simulink model "motor_position_ctrl"  (R2020b)
settings: Solver=ode15s  StartTime=0.0  StopTime=0.2  RelTol=1e-3  AbsTol=1e-7
undefined symbols (not defined in the file): Kd, Ki, Kp, N
settings Model: DataDictionary=motor_pos_data.sldd  Creator=ADMIN  LastModifiedBy=ADMIN

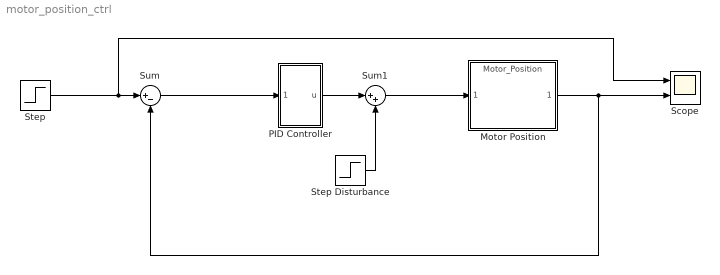
== system motor_position_ctrl ==
  "Motor Position " : ModelReference  ModelNameDialog=Motor_Position  ModelReferenceVersion=1.9
  PID Controller : Subsystem
  Scope : Scope  NumInputPorts=2
  Step : Step  Time=0  SampleTime=0
  Step Disturbance : Step  Time=0  SampleTime=0
  Sum : Sum  Inputs=|+-  SaturateOnIntegerOverflow=on
  Sum1 : Sum  Inputs=|++
  wires:
  Step/1 -> Scope/1, Sum/1
  "Motor Position "/1 -> Scope/2, Sum/2
  Sum/1 -> PID Controller/1(error)
  PID Controller/1(u) -> Sum1/1
  Sum1/1 -> "Motor Position "/1
  Step Disturbance/1 -> Sum1/2

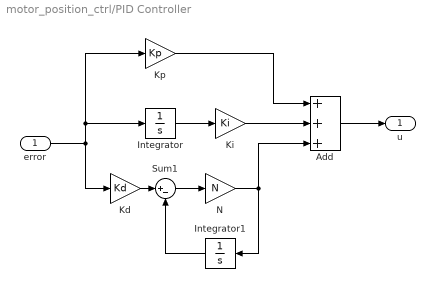
== system motor_position_ctrl/PID Controller ==
  error : Inport
  Add : Sum  Inputs=+++  SaturateOnIntegerOverflow=on
  Integrator : Integrator
  Integrator1 : Integrator
  Kd : Gain  Gain=Kd
  Ki : Gain  Gain=Ki
  Kp : Gain  Gain=Kp
  N : Gain  Gain=N
  Sum1 : Sum  Inputs=|+-
  u : Outport
  wires:
  error/1 -> Kp/1, Integrator/1, Kd/1
  Kd/1 -> Sum1/1
  Kp/1 -> Add/1
  Integrator/1 -> Ki/1
  Sum1/1 -> N/1
  Integrator1/1 -> Sum1/2
  Add/1 -> u/1
  N/1 -> Integrator1/1, Add/3
  Ki/1 -> Add/2
